simulink model "a"  (R2024b)
settings: Solver=VariableStepAuto  StartTime=0.0  StopTime=50  RelTol=1e-3
libraries: Solver_SF x1
settings Model: Creator=28677  LastModifiedBy=28677

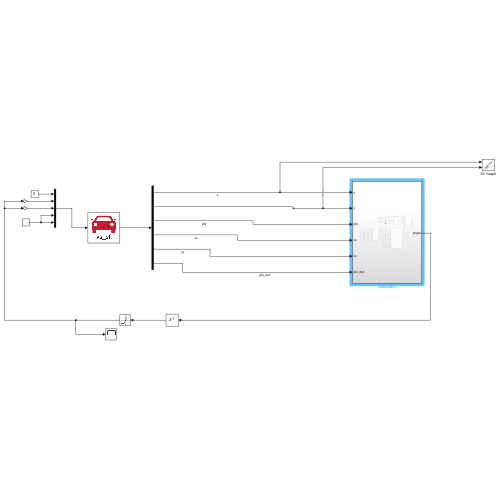
[thumbnail: Simulink's stored preview of the top-level diagram]
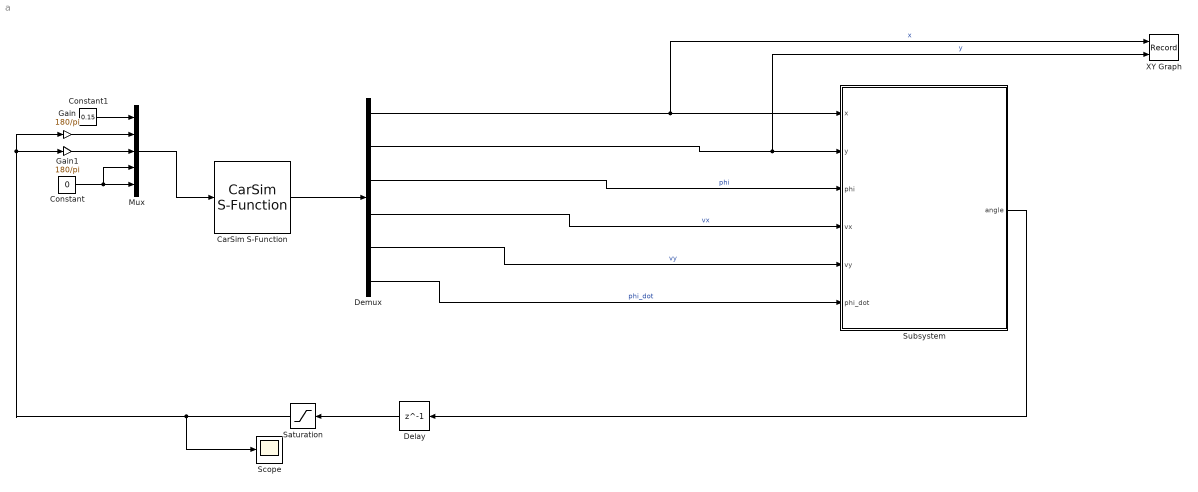
== system a ==
  CarSim S-Function : Solver_SF/CarSim S-Function  Priority=1  SIMFILE=simfile.sim  Run_RTs=off  vs_state_ind=Run  StopMode_ind=Vehicle Model
  Constant : Constant  Value=0
  Constant1 : Constant  Value=0.15
  Delay : Delay  DelayLength=1
  Demux : Demux  Outputs=6
  Gain : Gain  Gain=180/pi
  Gain1 : Gain  Gain=180/pi
  Mux : Mux  Inputs=5
  Saturation : Saturate  UpperLimit=1  LowerLimit=-1
  Scope : Scope
  Subsystem : Subsystem
  XY Graph : Record  FileSettingsInternal="{\"entries\":[{\"content\":{\"excelSettings\":{\"content\":{},\"type\":\"Streamout.ExcelSettings\"}},\"type\":\"Streamout.FileSettingStorage\",\"uuid\":\"\"}],\"packageUris\":[\"http:\\/\\/schema.mathworks.com\\/mf0\\/streamout_blocks\\/R2020a\"],\"version\":\"1.0\"}"  Layout=[1 1]  SignalsInternal="{\"entries\":[{\"content\":{\"signals\":[{\"content\":{\"blockPath\":[],\"dimensions\":[1],\"domain\":\"\",\"lineColor\":\"#a2142f\",\"plots\":[ 1 ],\"port\":1,\"sid\":[\"\"],\"signalID\":1,\"signalName\":\"x\"},\"type\":\"RecordBlkView.Signal\",\"uuid\":\"\"},{\"content\":{\"blockPath\":[],\"dimensions\":[1],\"domain\":\"\",\"lineColor\":\"#139fff\",\"plots\":[ 1 ],\"port\":2,\"sid\":[\"\"],\"signalID\":2,\"signalName\":\"y\"},\"type\":\"RecordBlkView.Signal\",\"uuid\":\"\"}]},\"type\":\"RecordBlkView.InputSignals\",\"uuid\":\"\"}],\"packageUris\":[\"http:\\/\\/schema.mathworks.com\\/mf0\\/streamout_blocks\\/R2020a\"],\"version\":\"1.0\"}"  VisualizationBindings="{\"xyplotplugin\":{\"info\":[{\"series\":[{\"bindingParametersList\":[{\"parameter\":\"X-Axis\",\"signalID\":1,\"signalName\":\"x\"},{\"parameter\":\"Y-Axis\",\"signalID\":2,\"signalName\":\"y\"}],\"seriesID\":0}],\"subplotID\":1}]}}"  CompatibilityTag=XY
  wires:
  CarSim S-Function/1 -> Demux/1
  Mux/1 -> CarSim S-Function/1
  Demux/1 -> XY Graph/1, Subsystem/1(x)  "x"
  Demux/2 -> XY Graph/2, Subsystem/2(y)  "y"
  Demux/3 -> Subsystem/3(phi)  "phi"
  Demux/4 -> Subsystem/4(vx)  "vx"
  Demux/5 -> Subsystem/5(vy)  "vy"
  Demux/6 -> Subsystem/6(phi_dot)  "phi_dot"
  Subsystem/1(angle) -> Delay/1
  Gain/1 -> Mux/2
  Gain1/1 -> Mux/3
  Delay/1 -> Saturation/1
  Constant/1 -> Mux/4, Mux/5
  Constant1/1 -> Mux/1
  Saturation/1 -> Scope/1, Gain/1, Gain1/1

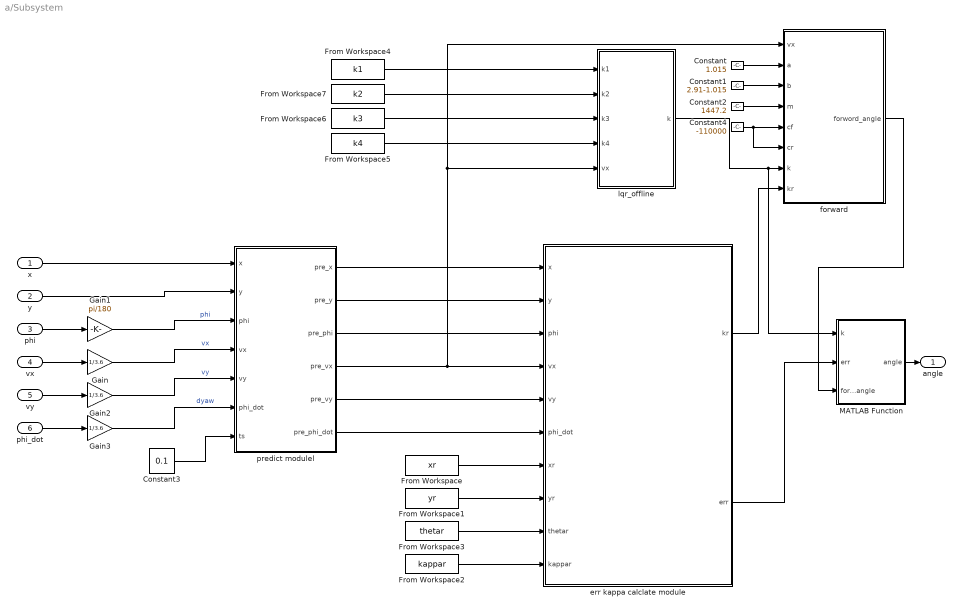
== system a/Subsystem ==
  x : Inport
  y : Inport  Port=2
  phi : Inport  Port=3
  vx : Inport  Port=4
  vy : Inport  Port=5
  phi_dot : Inport  Port=6
  Constant : Constant  Value=1.015
  Constant1 : Constant  Value=2.91-1.015
  Constant2 : Constant  Value=1447.2
  Constant3 : Constant  Value=0.1
  Constant4 : Constant  Value=-110000
  From Workspace : FromWorkspace  VariableName=xr
  From Workspace1 : FromWorkspace  VariableName=yr
  From Workspace2 : FromWorkspace  VariableName=kappar
  From Workspace3 : FromWorkspace  VariableName=thetar
  From Workspace4 : FromWorkspace  VariableName=k1
  From Workspace5 : FromWorkspace  VariableName=k4
  From Workspace6 : FromWorkspace  VariableName=k3
  From Workspace7 : FromWorkspace  VariableName=k2
  Gain : Gain  Gain=1/3.6
  Gain1 : Gain  Gain=pi/180
  Gain2 : Gain  Gain=1/3.6
  Gain3 : Gain  Gain=1/3.6
  MATLAB Function : MATLAB Function  TreatAsAtomicUnit=on
  err kappa calclate module : MATLAB Function  TreatAsAtomicUnit=on
  forward : MATLAB Function  TreatAsAtomicUnit=on
  lqr_offline : MATLAB Function  TreatAsAtomicUnit=on
  predict modulel : MATLAB Function  TreatAsAtomicUnit=on
  angle : Outport
  wires:
  lqr_offline/1(k) -> MATLAB Function/1(k), forward/7(k)
  predict modulel/6(pre_phi_dot) -> err kappa calclate module/6(phi_dot)
  predict modulel/4(pre_vx) -> forward/1(vx), lqr_offline/5(vx), err kappa calclate module/4(vx)
  Gain1/1 -> predict modulel/3(phi)  "phi"
  From Workspace2/1 -> err kappa calclate module/10(kappar)
  From Workspace/1 -> err kappa calclate module/7(xr)
  Gain3/1 -> predict modulel/6(phi_dot)  "dyaw"
  From Workspace3/1 -> err kappa calclate module/9(thetar)
  forward/1(forword_angle) -> MATLAB Function/3(forword_angle)
  Constant3/1 -> predict modulel/7(ts)
  From Workspace1/1 -> err kappa calclate module/8(yr)
  predict modulel/3(pre_phi) -> err kappa calclate module/3(phi)
  Gain/1 -> predict modulel/4(vx)  "vx"
  predict modulel/1(pre_x) -> err kappa calclate module/1(x)
  err kappa calclate module/2(err) -> MATLAB Function/2(err)
  Gain2/1 -> predict modulel/5(vy)  "vy"
  predict modulel/2(pre_y) -> err kappa calclate module/2(y)
  predict modulel/5(pre_vy) -> err kappa calclate module/5(vy)
  From Workspace4/1 -> lqr_offline/1(k1)
  y/1 -> predict modulel/2(y)
  err kappa calclate module/1(kr) -> forward/8(kr)
  phi/1 -> Gain1/1
  From Workspace5/1 -> lqr_offline/4(k4)
  From Workspace7/1 -> lqr_offline/2(k2)
  From Workspace6/1 -> lqr_offline/3(k3)
  phi_dot/1 -> Gain3/1
  vy/1 -> Gain2/1
  x/1 -> predict modulel/1(x)
  vx/1 -> Gain/1
  MATLAB Function/1(angle) -> angle/1
  Constant/1 -> forward/2(a)
  Constant1/1 -> forward/3(b)
  Constant2/1 -> forward/4(m)
  Constant4/1 -> forward/6(cr), forward/5(cf)

== matlab function a/Subsystem/err kappa calclate module ==
  data: x input; kr output; y input; phi input; vx input; vy input; phi_dot input; xr input; yr input; thetar input; kappar input; err output
function [kr,err] = fcn(x,y,phi,vx,vy,phi_dot,xr,yr,thetar,kappar)
n=length(xr);
d_min=(x-xr(1))^2+(y-yr(1))^2;
min=1;
for i=1:n
    d=(x-xr(i))^2+(y-yr(i))^2;
    if d<d_min
        d_min=d;
        min=i;
    end
end
dmin=min;
tor=[cos(thetar(dmin));sin(thetar(dmin))];
nor=[-sin(thetar(dmin));cos(thetar(dmin))];
d_err=[x-xr(dmin);y-yr(dmin)];
ed=nor'*d_err;
es=tor'*d_err;
%projection_point_thetar=thetar(dmin);apollo
projection_point_thetar=thetar(dmin)+kappar(dmin)*es;%apllo
ed_dot=vy*cos(phi-projection_point_thetar)+vx*sin(phi-projection_point_thetar);
%%%%%%%
ephi=sin(phi-projection_point_thetar);
%%%%%%%
s_dot=vx*cos(phi-projection_point_thetar)-vy*sin(phi-projection_point_thetar);
s_dot=s_dot/(1-kappar(dmin)*ed);
ephi_dot=phi_dot-kappar(dmin)*s_dot;
kr=kappar(dmin);
err=[ed;ed_dot;ephi;ephi_dot];

== matlab function a/Subsystem/predict modulel ==
  data: x input; pre_x output; pre_y output; pre_phi output; pre_vx output; pre_vy output; pre_phi_dot output; y input; phi input; vx input; vy input; phi_dot input; ts input
function [pre_x,pre_y,pre_phi,pre_vx,pre_vy,pre_phi_dot]  = fcn(x,y,phi,vx,vy,phi_dot,ts)
pre_x=x+vx*ts*cos(phi)-vy*ts*sin(phi);
pre_y=y+vy*ts*cos(phi)+vx*ts*sin(phi);
pre_phi=phi+phi_dot*ts;
pre_vx=vx;
pre_vy=vy;
pre_phi_dot=phi_dot;
end

== matlab function a/Subsystem/lqr_offline ==
  data: k1 input; k output; k2 input; k3 input; k4 input; vx input
function k = fcn(k1,k2,k3,k4,vx)
if abs(vx)<0.01
    k=[0,0,0,0];
else
    index=round(vx/0.01);
    k=[k1(index),k2(index),k3(index),k4(index)];
end
end

== matlab function a/Subsystem/forward ==
  data: vx input; a input; forword_angle output; b input; m input; cf input; cr input; k input; kr input
function forword_angle = fcn(vx,a,b,m,cf,cr,k,kr)
   forword_angle=kr*(a+b-b*k(3)-(m*vx*vx/(a+b))*((b/cf)+(a/cr)*k(3)-(a/cr)));
end

== matlab function a/Subsystem/MATLAB Function ==
  data: k input; angle output; err input; forword_angle input
function angle = fcn(k,err,forword_angle)

angle=-k*err+forword_angle;
end
